simulink model "kinEq_states_sim_Badweh"  (R2024a)
settings: Solver=FixedStepDiscrete  StartTime=0.0  StopTime=5  FixedStep=TS  RelTol=1e-3  EnableMultiTasking=on
PostLoadFcn:
  | params
model workspace (MAT data in the model file):
  Ia = 0.1
  Id = 0.25
  Pa = 5
  Pd = 9
  TS = 0.01
undefined symbols (not defined in the file): DiscIntNeverNeededParam, L, r, StartTheta, StartX, StartY
libraries: simulink_extras x3, slpidlib x2
settings Model: Creator=mgovinda  LastModifiedBy=Sheen
settings SolverCC: AlgebraicLoopSolver=TrustRegion
settings DataIOCC: LimitDataPoints=on  SaveFormat=Array  ReturnWorkspaceOutputs=off
settings OptimizationCC: LifeSpan=inf
settings DebuggingCC: UnderspecifiedInitializationDetection=Classic  MergeDetectMultiDrivingBlocksExec=none  UnconnectedInputMsg=warning  UnconnectedOutputMsg=warning  UnconnectedLineMsg=warning  SFUnexpectedBacktrackingDiag=warning  SFNoUnconditionalDefaultTransitionDiag=warning  SFExecutionAtInitializationDiag=none  ArithmeticOperatorsInVariantConditions=warning
settings HardwareCC: ProdBitPerPointer=32  ProdBitPerSizeT=32  ProdBitPerPtrDiffT=32  ProdLargestAtomicFloat=None  ProdIntDivRoundTo=Undefined  ProdEndianess=Unspecified  ProdWordSize=32  ProdHWDeviceType=32-bit Generic
settings ModelReferenceCC: EnableRefExpFcnMdlSchedulingChecks=on  PropagateSignalLabelsOutOfModel=off
settings SFSimCC: SimUseLocalCustomCode=off  CustomCodeUndefinedFunction=UseInterfaceOnly
settings RTWCC: RTWUseLocalCustomCode=off  GPUComputeCapability=3.5
settings CodeAppCC: StateflowObjectComments=on
settings GRTTargetCC: TargetLangStandard=C89/C90 (ANSI)
settings ConfigComp: CovMetricSettings=dw  CovSaveCumulativeToWorkspaceVar=on  CovSaveSingleToWorkspaceVar=on  CovExternalEMLEnable=off

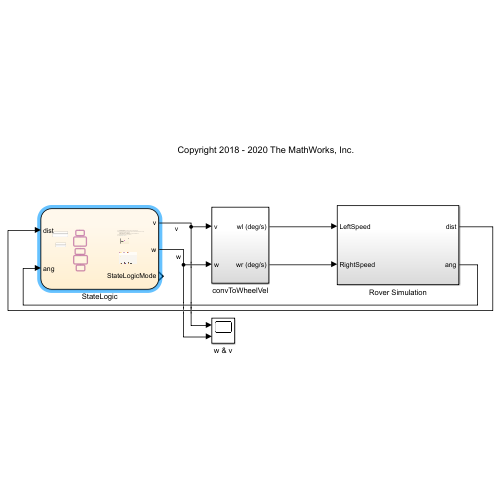
[thumbnail: Simulink's stored preview of the top-level diagram]
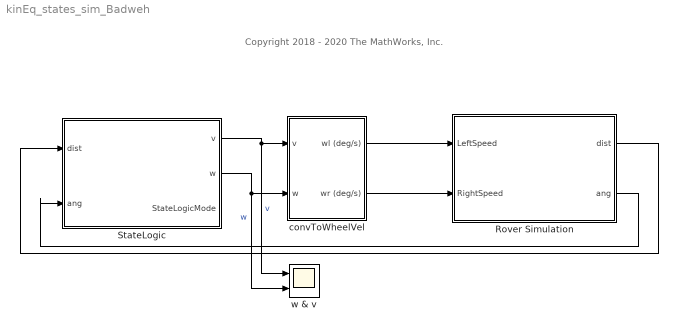
== system kinEq_states_sim_Badweh ==
  note: Copyright 2018 - 2020 The MathWorks, Inc.
  Rover Simulation : Subsystem
  StateLogic : Stateflow chart  TreatAsAtomicUnit=on
  convToWheelVel : Subsystem
  w & v : Scope  NumInputPorts=2
  wires:
  StateLogic/1(v) -> w & v/1, convToWheelVel/1(v)  "v"
  StateLogic/2(w) -> w & v/2, convToWheelVel/2(w)  "w"
  Rover Simulation/1(dist) -> StateLogic/1(dist)
  Rover Simulation/2(ang) -> StateLogic/2(ang)
  convToWheelVel/1(wl (deg/s)) -> Rover Simulation/1(LeftSpeed)
  convToWheelVel/2(wr (deg/s)) -> Rover Simulation/2(RightSpeed)

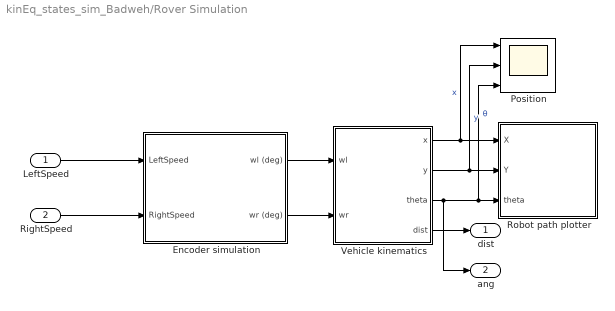
== system kinEq_states_sim_Badweh/Rover Simulation ==
  LeftSpeed : Inport
  RightSpeed : Inport  Port=2
  " Encoder simulation" : Subsystem
  Position : Scope  NumInputPorts=3
  Robot path plotter : Subsystem
  "Vehicle kinematics " : Subsystem
  dist : Outport  VectorParamsAs1DForOutWhenUnconnected=off
  ang : Outport  Port=2  VectorParamsAs1DForOutWhenUnconnected=off
  wires:
  "Vehicle kinematics "/1(x) -> Position/1, Robot path plotter/1(X)  "x"
  "Vehicle kinematics "/2(y) -> Position/2, Robot path plotter/2(Y)  "y"
  "Vehicle kinematics "/3(theta) -> ang/1, Position/3, Robot path plotter/3(theta)  "θ"
  LeftSpeed/1 -> " Encoder simulation"/1(LeftSpeed)
  RightSpeed/1 -> " Encoder simulation"/2(RightSpeed)
  " Encoder simulation"/1(wl (deg)) -> "Vehicle kinematics "/1(wl)
  " Encoder simulation"/2(wr (deg)) -> "Vehicle kinematics "/2(wr)
  "Vehicle kinematics "/4(dist) -> dist/1

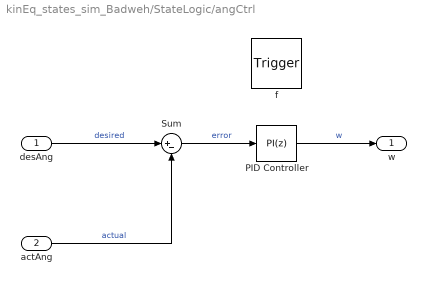
== system kinEq_states_sim_Badweh/StateLogic/angCtrl ==
  desAng : Inport  OutDataTypeStr=double  PortDimensions=1
  actAng : Inport  Port=2  OutDataTypeStr=double  PortDimensions=1
  f : TriggerPort  TriggerType=function-call  VariantControl=(inherit)
      settings: CopyFcn=Stateflow.SLINSF.SimulinkMan.removeBlockPreDeleteFcn  PreDeleteFcn=Stateflow.SLINSF.SimulinkMan.unsafePredeleteFcn
  PID Controller : slpidlib/PID Controller  Controller=PI  Form=Parallel  TimeDomain=Discrete-time  UseExternalTs=off  SampleTime=-1  IntegratorMethod=Forward Euler  FilterMethod=Forward Euler  ControllerParametersSource=internal  P=1.2  I=0.2  UseKiTs=off  D=0  UseExternalDerivativeSource=off  N=100  UseFilter=on  TunerSelectOption=Transfer Function Based (PID Tuner App)  InitialConditionSource=internal  InitialConditionForIntegrator=0  InitialConditionForFilter=0  DifferentiatorICPrevScaledInput=0  ExternalReset=none  TrackingMode=off  Kt=1  LimitOutput=off  SatLimitsSource=internal  UpperSaturationLimit=inf  LowerSaturationLimit=-inf  LinearizeAsGain=on  AntiWindupMode=none  Kb=1  LimitIntegrator=off  UpperIntegratorSaturationLimit=inf  LowerIntegratorSaturationLimit=-inf  POutMin=[]  POutMax=[]  IOutMin=[]  IOutMax=[]  DOutMin=[]  DOutMax=[]  NOutMin=[]  NOutMax=[]  SumOutMin=[]  SumOutMax=[]  SaturationOutMin=[]  SaturationOutMax=[]  PParamMin=[]  PParamMax=[]  IParamMin=[]  IParamMax=[]  DParamMin=[]  DParamMax=[]  NParamMin=[]  NParamMax=[]  KbParamMin=[]  KbParamMax=[]  KtParamMin=[]  KtParamMax=[]  KbOutMin=[]  KbOutMax=[]  KtOutMin=[]  KtOutMax=[]  IntegratorOutMin=[]  IntegratorOutMax=[]  FilterOutMin=[]  FilterOutMax=[]  SumI1OutMin=[]  SumI1OutMax=[]  SumI2OutMin=[]  SumI2OutMax=[]  SumI3OutMin=[]  SumI3OutMax=[]  SumI4OutMin=[]  SumI4OutMax=[]  SumDOutMin=[]  SumDOutMax=[]  DifferentiatorOutMin=[]  DifferentiatorOutMax=[]  FilterDiffOutCoefMin=[]  FilterDiffOutCoefMax=[]  ReciprocalOutMin=[]  ReciprocalOutMax=[]  SumDenOutMin=[]  SumDenOutMax=[]  SumNumOutMin=[]  SumNumOutMax=[]  DivideOutMin=[]  DivideOutMax=[]  UdiffTsProdOutMin=[]  UdiffTsProdOutMax=[]  NTsProdOutMin=[]  NTsProdOutMax=[]  UintegralTsProdOutMin=[]  UintegralTsProdOutMax=[]  UngainTsProdOutMin=[]  UngainTsProdOutMax=[]  ClampingZeroOutDataTypeStr=Inherit: Inherit via back propagation  ClampingZeroOutMin=[]  ClampingZeroOutMax=[]  FilterDenConstantOutDataTypeStr=Inherit: Inherit via back propagation  FilterDenConstantOutMin=[]  FilterDenConstantOutMax=[]  PCopyOutDataTypeStr=Inherit: Inherit via back propagation  PCopyOutMin=[]  PCopyOutMax=[]  NCopyOutDataTypeStr=Inherit: Inherit via back propagation  NCopyOutMin=[]  NCopyOutMax=[]  IntegratorContinuousStateAttributes=''  IntegratorStateMustResolveToSignalObject=off  IntegratorRTWStateStorageClass=Auto  FilterContinuousStateAttributes=''  FilterStateMustResolveToSignalObject=off  FilterRTWStateStorageClass=Auto  ParallelPVariant=InternalParameters  IdealPVariant=Disabled  IVariant=InternalParameters  DVariant=Disabled  IntegratorVariant=Discrete  SatVariant=Disabled  AWVariant=Passthrough  PCopyVariant=Disabled  TRVariant=Disabled  FdbkBlocksVariant=Forward  IdealPFdbkVariant=Disabled  SatFdbkVariant=Disabled  DerivativeFilterVariant=Disabled  NVariant=Disabled  NCopyVariant=Disabled_SignalSpec  FilterICVariant=Disabled  IntegratorICVariant=InternalICs  ExternalResetVariant=Disabled  TRSumVariant=Passthrough  SumFdbkVariant=Disabled  SumVariant=Sum_PI  TsampFilterVariant=InternalTs  TsampNgainVariant=Passthrough  TsampIntegralVariant=Disabled_SignalSpec  ExternalSaturationOutDataTypeStr=Inherit: Same as second input  DerivativeSourceVariant=Disabled
  Sum : Sum  Inputs=|+-
  w : Outport  VectorParamsAs1DForOutWhenUnconnected=off
  wires:
  actAng/1 -> Sum/2  "actual"
  desAng/1 -> Sum/1  "desired"
  PID Controller/1 -> w/1  "w"
  Sum/1 -> PID Controller/1  "error"

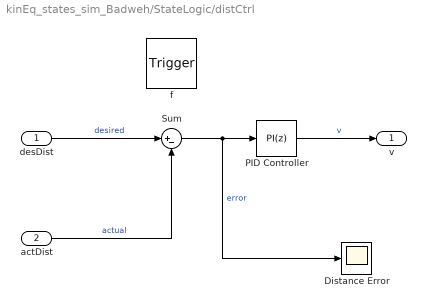
== system kinEq_states_sim_Badweh/StateLogic/distCtrl ==
  desDist : Inport  OutDataTypeStr=double  PortDimensions=1
  actDist : Inport  Port=2  OutDataTypeStr=double  PortDimensions=1
  f : TriggerPort  TriggerType=function-call  VariantControl=(inherit)
      settings: CopyFcn=Stateflow.SLINSF.SimulinkMan.removeBlockPreDeleteFcn  PreDeleteFcn=Stateflow.SLINSF.SimulinkMan.unsafePredeleteFcn
  Distance Error : Scope
  PID Controller : slpidlib/PID Controller  Controller=PI  Form=Parallel  TimeDomain=Discrete-time  UseExternalTs=off  SampleTime=-1  IntegratorMethod=Forward Euler  FilterMethod=Forward Euler  ControllerParametersSource=internal  P=0.25  I=0.05  UseKiTs=off  D=0  UseExternalDerivativeSource=off  N=100  UseFilter=on  TunerSelectOption=Transfer Function Based (PID Tuner App)  InitialConditionSource=internal  InitialConditionForIntegrator=0  InitialConditionForFilter=0  DifferentiatorICPrevScaledInput=0  ExternalReset=none  TrackingMode=off  Kt=1  LimitOutput=off  SatLimitsSource=internal  UpperSaturationLimit=inf  LowerSaturationLimit=-inf  LinearizeAsGain=on  AntiWindupMode=none  Kb=1  LimitIntegrator=off  UpperIntegratorSaturationLimit=inf  LowerIntegratorSaturationLimit=-inf  POutMin=[]  POutMax=[]  IOutMin=[]  IOutMax=[]  DOutMin=[]  DOutMax=[]  NOutMin=[]  NOutMax=[]  SumOutMin=[]  SumOutMax=[]  SaturationOutMin=[]  SaturationOutMax=[]  PParamMin=[]  PParamMax=[]  IParamMin=[]  IParamMax=[]  DParamMin=[]  DParamMax=[]  NParamMin=[]  NParamMax=[]  KbParamMin=[]  KbParamMax=[]  KtParamMin=[]  KtParamMax=[]  KbOutMin=[]  KbOutMax=[]  KtOutMin=[]  KtOutMax=[]  IntegratorOutMin=[]  IntegratorOutMax=[]  FilterOutMin=[]  FilterOutMax=[]  SumI1OutMin=[]  SumI1OutMax=[]  SumI2OutMin=[]  SumI2OutMax=[]  SumI3OutMin=[]  SumI3OutMax=[]  SumI4OutMin=[]  SumI4OutMax=[]  SumDOutMin=[]  SumDOutMax=[]  DifferentiatorOutMin=[]  DifferentiatorOutMax=[]  FilterDiffOutCoefMin=[]  FilterDiffOutCoefMax=[]  ReciprocalOutMin=[]  ReciprocalOutMax=[]  SumDenOutMin=[]  SumDenOutMax=[]  SumNumOutMin=[]  SumNumOutMax=[]  DivideOutMin=[]  DivideOutMax=[]  UdiffTsProdOutMin=[]  UdiffTsProdOutMax=[]  NTsProdOutMin=[]  NTsProdOutMax=[]  UintegralTsProdOutMin=[]  UintegralTsProdOutMax=[]  UngainTsProdOutMin=[]  UngainTsProdOutMax=[]  ClampingZeroOutDataTypeStr=Inherit: Inherit via back propagation  ClampingZeroOutMin=[]  ClampingZeroOutMax=[]  FilterDenConstantOutDataTypeStr=Inherit: Inherit via back propagation  FilterDenConstantOutMin=[]  FilterDenConstantOutMax=[]  PCopyOutDataTypeStr=Inherit: Inherit via back propagation  PCopyOutMin=[]  PCopyOutMax=[]  NCopyOutDataTypeStr=Inherit: Inherit via back propagation  NCopyOutMin=[]  NCopyOutMax=[]  IntegratorContinuousStateAttributes=''  IntegratorStateMustResolveToSignalObject=off  IntegratorRTWStateStorageClass=Auto  FilterContinuousStateAttributes=''  FilterStateMustResolveToSignalObject=off  FilterRTWStateStorageClass=Auto  ParallelPVariant=InternalParameters  IdealPVariant=Disabled  IVariant=InternalParameters  DVariant=Disabled  IntegratorVariant=Discrete  SatVariant=Disabled  AWVariant=Passthrough  PCopyVariant=Disabled  TRVariant=Disabled  FdbkBlocksVariant=Forward  IdealPFdbkVariant=Disabled  SatFdbkVariant=Disabled  DerivativeFilterVariant=Disabled  NVariant=Disabled  NCopyVariant=Disabled_SignalSpec  FilterICVariant=Disabled  IntegratorICVariant=InternalICs  ExternalResetVariant=Disabled  TRSumVariant=Passthrough  SumFdbkVariant=Disabled  SumVariant=Sum_PI  TsampFilterVariant=InternalTs  TsampNgainVariant=Passthrough  TsampIntegralVariant=Disabled_SignalSpec  ExternalSaturationOutDataTypeStr=Inherit: Same as second input  DerivativeSourceVariant=Disabled
  Sum : Sum  Inputs=|+-
  v : Outport  VectorParamsAs1DForOutWhenUnconnected=off
  wires:
  actDist/1 -> Sum/2  "actual"
  desDist/1 -> Sum/1  "desired"
  PID Controller/1 -> v/1  "v"
  Sum/1 -> Distance Error/1, PID Controller/1  "error"

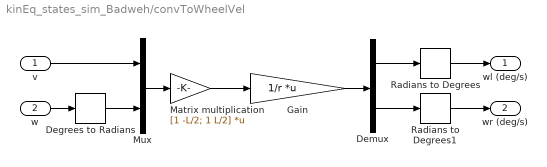
== system kinEq_states_sim_Badweh/convToWheelVel ==
  v : Inport
  w : Inport  Port=2
  " Gain" : Gain  Gain=1/r  Multiplication=Matrix(K*u)
  Degrees to Radians : simulink_extras/Transformations/Degrees to Radians
  Demux : Demux  Outputs=2
  Matrix multiplication : Gain  Gain=[1 -L/2; 1 L/2]  Multiplication=Matrix(K*u)
  Mux : Mux  Inputs=2
  Radians to Degrees : simulink_extras/Transformations/Radians to Degrees
  Radians to Degrees1 : simulink_extras/Transformations/Radians to Degrees
  wl (deg/s) : Outport  VectorParamsAs1DForOutWhenUnconnected=off
  wr (deg/s) : Outport  Port=2  VectorParamsAs1DForOutWhenUnconnected=off
  wires:
  " Gain"/1 -> Demux/1
  Matrix multiplication/1 -> " Gain"/1
  v/1 -> Mux/1
  Mux/1 -> Matrix multiplication/1
  Demux/1 -> Radians to Degrees/1
  Demux/2 -> Radians to Degrees1/1
  w/1 -> Degrees to Radians/1
  Radians to Degrees/1 -> wl (deg/s)/1
  Radians to Degrees1/1 -> wr (deg/s)/1
  Degrees to Radians/1 -> Mux/2

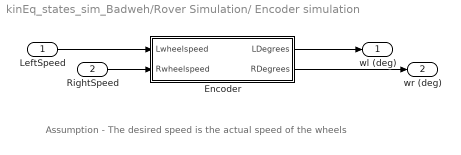
== system kinEq_states_sim_Badweh/Rover Simulation/ Encoder simulation ==
  note: Assumption - The desired speed is the actual speed of the wheels
  LeftSpeed : Inport
  RightSpeed : Inport  Port=2
  Encoder : Subsystem
  wl (deg) : Outport  VectorParamsAs1DForOutWhenUnconnected=off
  wr (deg) : Outport  Port=2  VectorParamsAs1DForOutWhenUnconnected=off
  wires:
  Encoder/1(LDegrees) -> wl (deg)/1
  Encoder/2(RDegrees) -> wr (deg)/1
  RightSpeed/1 -> Encoder/2(Rwheelspeed)
  LeftSpeed/1 -> Encoder/1(Lwheelspeed)

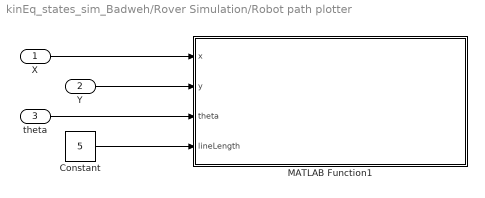
== system kinEq_states_sim_Badweh/Rover Simulation/Robot path plotter ==
  X : Inport
  Y : Inport  Port=2
  theta : Inport  Port=3
  Constant : Constant  Value=5
  MATLAB Function1 : MATLAB Function  TreatAsAtomicUnit=on
  wires:
  Constant/1 -> MATLAB Function1/4(lineLength)
  X/1 -> MATLAB Function1/1(x)
  Y/1 -> MATLAB Function1/2(y)
  theta/1 -> MATLAB Function1/3(theta)

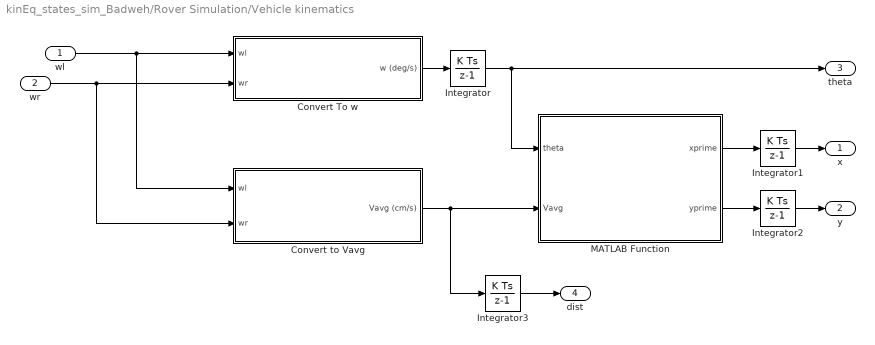
== system kinEq_states_sim_Badweh/Rover Simulation/Vehicle kinematics  ==
  wl : Inport
  wr : Inport  Port=2
  Convert To w : Subsystem
  Convert to Vavg : Subsystem
  Integrator : DiscreteIntegrator  gainval=1  InitialCondition=StartTheta  SampleTime=-1  ICPrevOutput=DiscIntNeverNeededParam  ICPrevScaledInput=DiscIntNeverNeededParam
  Integrator1 : DiscreteIntegrator  gainval=1  InitialCondition=StartX  SampleTime=-1  ICPrevOutput=DiscIntNeverNeededParam  ICPrevScaledInput=DiscIntNeverNeededParam
  Integrator2 : DiscreteIntegrator  gainval=1  InitialCondition=StartY  SampleTime=-1  ICPrevOutput=DiscIntNeverNeededParam  ICPrevScaledInput=DiscIntNeverNeededParam
  Integrator3 : DiscreteIntegrator  gainval=1  SampleTime=-1  ICPrevOutput=DiscIntNeverNeededParam  ICPrevScaledInput=DiscIntNeverNeededParam
  MATLAB Function : MATLAB Function  TreatAsAtomicUnit=on
  x : Outport  VectorParamsAs1DForOutWhenUnconnected=off
  y : Outport  Port=2  VectorParamsAs1DForOutWhenUnconnected=off
  theta : Outport  Port=3  VectorParamsAs1DForOutWhenUnconnected=off
  dist : Outport  Port=4  VectorParamsAs1DForOutWhenUnconnected=off
  wires:
  MATLAB Function/1(xprime) -> Integrator1/1
  MATLAB Function/2(yprime) -> Integrator2/1
  Integrator1/1 -> x/1
  Integrator2/1 -> y/1
  Integrator/1 -> theta/1, MATLAB Function/1(theta)
  wl/1 -> Convert to Vavg/1(wl), Convert To w/1(wl)
  wr/1 -> Convert to Vavg/2(wr), Convert To w/2(wr)
  Convert to Vavg/1(Vavg (cm/s)) -> Integrator3/1, MATLAB Function/2(Vavg)
  Convert To w/1(w (deg/s)) -> Integrator/1
  Integrator3/1 -> dist/1

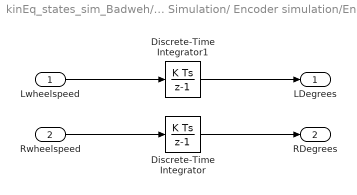
== system kinEq_states_sim_Badweh/Rover Simulation/ Encoder simulation/Encoder ==
  Lwheelspeed : Inport
  Rwheelspeed : Inport  Port=2
  Discrete-Time Integrator : DiscreteIntegrator  SampleTime=-1  ICPrevOutput=DiscIntNeverNeededParam  ICPrevScaledInput=DiscIntNeverNeededParam
  Discrete-Time Integrator1 : DiscreteIntegrator  SampleTime=-1  ICPrevOutput=DiscIntNeverNeededParam  ICPrevScaledInput=DiscIntNeverNeededParam
  LDegrees : Outport  VectorParamsAs1DForOutWhenUnconnected=off
  RDegrees : Outport  Port=2  VectorParamsAs1DForOutWhenUnconnected=off
  wires:
  Rwheelspeed/1 -> Discrete-Time Integrator/1
  Lwheelspeed/1 -> Discrete-Time Integrator1/1
  Discrete-Time Integrator/1 -> RDegrees/1
  Discrete-Time Integrator1/1 -> LDegrees/1

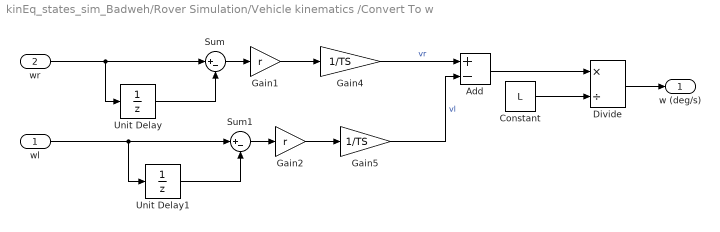
== system kinEq_states_sim_Badweh/Rover Simulation/Vehicle kinematics /Convert To w ==
  wl : Inport
  wr : Inport  Port=2
  Add : Sum  Inputs=+-
  Constant : Constant  Value=L
  Divide : Product  Inputs=*/
  Gain1 : Gain  Gain=r
  Gain2 : Gain  Gain=r
  Gain4 : Gain  Gain=1/TS
  Gain5 : Gain  Gain=1/TS
  Sum : Sum  Inputs=|+-
  Sum1 : Sum  Inputs=|+-
  Unit Delay : UnitDelay  SampleTime=-1  HasFrameUpgradeWarning=on
  Unit Delay1 : UnitDelay  SampleTime=-1  HasFrameUpgradeWarning=on
  w (deg/s) : Outport  VectorParamsAs1DForOutWhenUnconnected=off
  wires:
  Unit Delay1/1 -> Sum1/2
  Sum1/1 -> Gain2/1
  wl/1 -> Unit Delay1/1, Sum1/1
  wr/1 -> Sum/1, Unit Delay/1
  Sum/1 -> Gain1/1
  Unit Delay/1 -> Sum/2
  Gain1/1 -> Gain4/1
  Gain2/1 -> Gain5/1
  Add/1 -> Divide/1
  Constant/1 -> Divide/2
  Gain4/1 -> Add/1  "vr"
  Gain5/1 -> Add/2  "vl"
  Divide/1 -> w (deg/s)/1

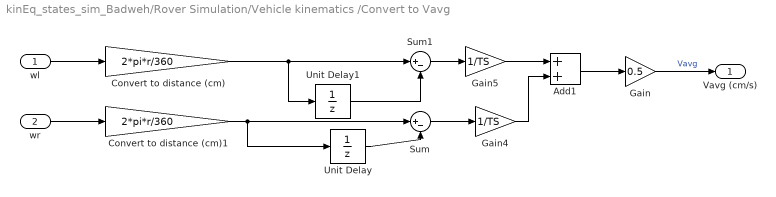
== system kinEq_states_sim_Badweh/Rover Simulation/Vehicle kinematics /Convert to Vavg ==
  wl : Inport
  wr : Inport  Port=2
  Add1 : Sum
  Convert to distance (cm) : Gain  Gain=2*pi*r/360
  Convert to distance (cm)1 : Gain  Gain=2*pi*r/360
  Gain : Gain  Gain=0.5
  Gain4 : Gain  Gain=1/TS
  Gain5 : Gain  Gain=1/TS
  Sum : Sum  Inputs=|+-
  Sum1 : Sum  Inputs=|+-
  Unit Delay : UnitDelay  SampleTime=-1  HasFrameUpgradeWarning=on
  Unit Delay1 : UnitDelay  SampleTime=-1  HasFrameUpgradeWarning=on
  Vavg (cm/s) : Outport  VectorParamsAs1DForOutWhenUnconnected=off
  wires:
  Gain/1 -> Vavg (cm/s)/1  "Vavg"
  Add1/1 -> Gain/1
  Unit Delay/1 -> Sum/2
  Sum/1 -> Gain4/1
  wr/1 -> Convert to distance (cm)1/1
  Gain4/1 -> Add1/2
  Gain5/1 -> Add1/1
  Sum1/1 -> Gain5/1
  Unit Delay1/1 -> Sum1/2
  wl/1 -> Convert to distance (cm)/1
  Convert to distance (cm)/1 -> Unit Delay1/1, Sum1/1
  Convert to distance (cm)1/1 -> Unit Delay/1, Sum/1

== matlab function kinEq_states_sim_Badweh/Rover Simulation/Vehicle kinematics /MATLAB Function ==
  settings: updateMethod=DISCRETE  sampleTime=TS
  data: xprime output; yprime output; theta input; Vavg input
function [xprime, yprime] = vehiclesPath(theta, Vavg)
%#codegen

% Implement the equation for the real-world location of the rover
xprime = Vavg*cosd(theta);
yprime = Vavg*sind(theta);

== stateflow chart kinEq_states_sim_Badweh/StateLogic ==
  note: State (Block)
      | Transition Condition (->)
      | 	Tested at every time step denoted by the sample time
  note: Entry : executed immediatley upon entering the state. It run before anything else
      | Thought of it as setup
      | During: Execute after 'Entry'. It stays executing as long as the state is still activate. Think of it as 'for' loop
      | both the during and exit actions set
      | velocity, v = PI control %% Slow down as we reaches the desire distance
      | angular velocity, w = 0 %% No turning
      | Sumulink function distCtrl() is called at every time step
      |
      | Exit: when abs(desDist - dist) < 0.1
  state StopFirst
    entry:
    v = 0; w= 0;
  note: Simulation Begin at 'StopFirst'
      | set
      | v = 0
      | w = 0
  state v = distCtrl(desDist,actDist) [function]
  note: [] Learn to debug the Stateflow
  state MoveForward
    entry:
    desDist = 30;
    during, exit:
    v = distCtrl(desDist,dist);
    w = 0;
  note: ?
  note: Set velocity at constant
      | 	v = 10
      | 	w = 90
  state w = angCtrl(desAng,actAng) [function]
  state Pause
    entry:
    v = 0;
    w = 0;
  note: ?
  state Turn
    entry:
    desAng = 180;
    during, exit:
    v = 0;
    w = angCtrl(desAng,ang);
  state Stop
    entry:
    v = 0;
    w = 0;
  (default) -> StopFirst
  StopFirst -> MoveForward : after(1,sec)
  MoveForward -> Pause : [abs(desDist - dist) < 0.1]
  Pause -> Turn : after(1,sec)
  Turn -> Stop : [abs(desAng - ang) < 0.1]
  data: desDist function_input double size=1; actDist function_input double size=1; v function_output; desAng function_input double size=1; actAng function_input double size=1; w function_output; dist input; ang input; v output; w output; desDist local; desAng local; StateLogicMode output Enum: StateLogicModeType

== matlab function kinEq_states_sim_Badweh/Rover Simulation/Robot path plotter/MATLAB Function1 ==
  data: x input; y input; theta input; lineLength input; StartX parameter; StartY parameter; StartTheta parameter
function plotRobot(x,y,theta,lineLength, StartX, StartY, StartTheta)

% Create persistent variables for the figure windows
persistent h h1 h2;

if isempty(h)
    % Set up the initial figure window to display the initial position of
    % the rover
    h = figure('name','Map of the Robot');
    h1 = plot(StartX,StartY,'bo');
    hold on
    xlim([0 100])
    ylim([0 100])
    
    % Update the plot to show the heading of the rover
    xp = [StartX StartX+lineLength*cosd(StartTheta)];
    yp = [StartY StartY+lineLength*sind(StartTheta)];
    h2 = plot(xp,yp,'b');
    hold off
end

% Visualize the rover's path and heading
set(h1,'xdata',x,'ydata',y)
xp = [x x+lineLength*cosd(theta)];
yp = [y y+lineLength*sind(theta)];
set(h2,'xdata',xp,'ydata',yp)
drawnow('limitrate')
